simulink model "P_simple_sim_non_linear_model"  (R2015b)
settings: Solver=FixedStepAuto  StartTime=0.0  StopTime=t_f  FixedStep=0.005  RelTol=1e-3
values from neighbouring files (symbols this model uses):
  a = 0.3    [ICPtesting.m]    (also in LQR_controller_development.m = 0.0165; LQR_controller_development_new.m = 0.0165; RotationMatrixProperties.m; controller_params.m = 0.0165)
  b = 20*pi/180    (= 0.349065850399)    [LQR_controller_development.m]    (also in LQR_controller_development_new.m; RotationMatrixProperties.m = 0.3; controller_params.m)
  bp = 0.6    [LQR_controller_development.m]    (also in LQR_controller_development_new.m = 0.03; controller_params.m = 0.84111335)
  br = 0.3    [LQR_controller_development.m]    (also in LQR_controller_development_new.m = 0.03; controller_params.m = 0.246502067333)
  bw = 0.6    [LQR_controller_development.m]    (also in LQR_controller_development_new.m = 0.03; controller_params.m = 0.377213737333)
  bx = 10    [LQR_controller_development.m]    (also in LQR_controller_development_new.m = 12; controller_params.m = 7.95)
  by = 20    [LQR_controller_development.m]    (also in LQR_controller_development_new.m = 16; controller_params.m = 22.75)
  bz = 20    [LQR_controller_development.m]    (also in LQR_controller_development_new.m = 18; controller_params.m = 37.1)
  c = double(solve(cos(c_sym)*a-sin(c_sym)*lbx == 0,c_sym))    [LQR_controller_development.m]    (also in LQR_controller_development_new.m; RotationMatrixProperties.m = 0.3; controller_params.m = 8)
  dt = 0.02    [LQR_controller_development.m]    (also in LQR_controller_development_new.m = 0.05; controller_params.m = 0.05)
  Ixx = 0.015    [LQR_controller_development.m]    (also in LQR_controller_development_new.m; controller_params.m = 0.0098)
  Iyy = 0.035    [LQR_controller_development.m]    (also in LQR_controller_development_new.m; controller_params.m = 0.075)
  Izz = 0.035    [LQR_controller_development.m]    (also in LQR_controller_development_new.m; controller_params.m = 0.08)
  Kd = round(Kd,4)    [LQI_controller_development.m]    (also in LQR_controller_development.m; LQR_controller_development_new.m)
  lax = 0.15    [LQR_controller_development.m]    (also in LQR_controller_development_new.m; controller_params.m = 0.2)
  lay = 0.1    [LQR_controller_development.m]    (also in LQR_controller_development_new.m; controller_params.m)
  lbx = 0.12    [LQR_controller_development.m]    (also in LQR_controller_development_new.m; controller_params.m = 0.175)
  m = m*1.2    [LQI_controller_development.m]    (also in LQR_controller_development.m = 3; LQR_controller_development_new.m = 4; controller_params.m = 3.8)
  Tp_deadband = 0.2    [LQR_controller_development.m]    (also in LQR_controller_development_new.m = 0.1; controller_params.m = 0.05)
  Tp_min_input = 0.5    [LQR_controller_development.m]    (also in LQR_controller_development_new.m = 0.2; controller_params.m = 0.1)
  TpL = -140    [LQR_controller_development.m]    (also in LQR_controller_development_new.m = -22; controller_params.m = -8)
  TpU = 160    [LQR_controller_development.m]    (also in LQR_controller_development_new.m = 25; controller_params.m = 8)
  Ts_deadband = 0.2    [LQR_controller_development.m]    (also in LQR_controller_development_new.m = 0.1; controller_params.m = 0.05)
  Ts_min_input = 0.5    [LQR_controller_development.m]    (also in LQR_controller_development_new.m = 0.2; controller_params.m = 0.1)
  TsL = -70    [LQR_controller_development.m]    (also in LQR_controller_development_new.m = -14; controller_params.m = -4)
  TsU = 80    [LQR_controller_development.m]    (also in LQR_controller_development_new.m = 15; controller_params.m = 4)
undefined symbols (not defined in the file or in its folder): DiscIntNeverNeededParam
settings Model: Creator=meskupie  LastModifiedBy=meskupie

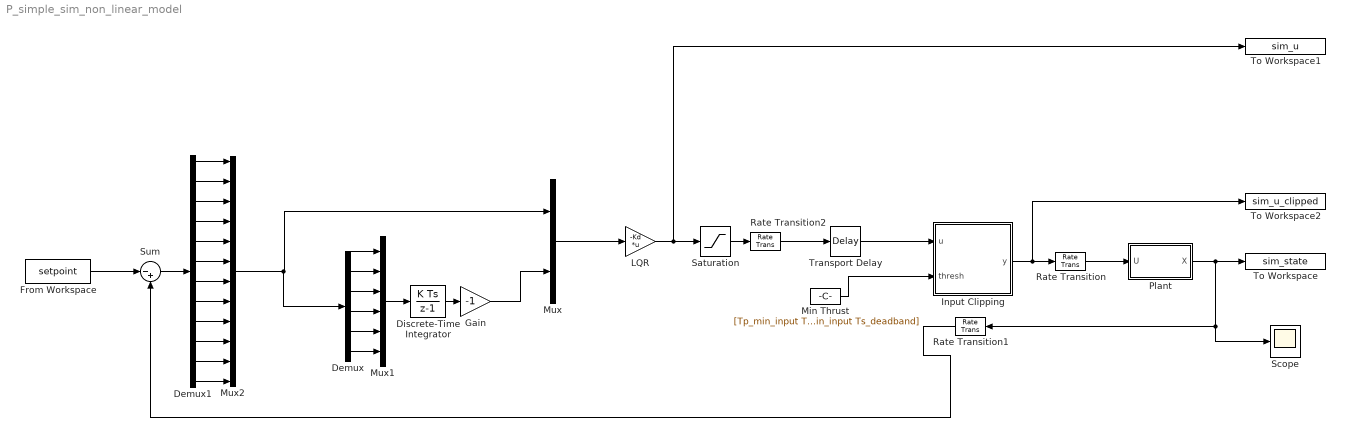
== system P_simple_sim_non_linear_model ==
  Demux : Demux  Outputs=12
  Demux1 : Demux  Outputs=12
  Discrete-Time Integrator : DiscreteIntegrator  InitialConditionSetting=State (most efficient)  SampleTime=dt  ICPrevOutput=DiscIntNeverNeededParam  ICPrevScaledInput=DiscIntNeverNeededParam
  From Workspace : FromWorkspace  VariableName=setpoint  SampleTime=dt
  Gain : Gain  Gain=-1
  Input Clipping : MATLAB Function  TreatAsAtomicUnit=on
  LQR : Gain  Gain=-Kd  Multiplication=Matrix(K*u)
  Min Thrust : Constant  Value=[Tp_min_input Tp_deadband Ts_min_input Ts_deadband]  SampleTime=-1
  Mux : Mux  Inputs=2
  Mux1 : Mux  Inputs=6
  Mux2 : Mux  Inputs=12
  Plant : Subsystem
  Rate Transition : RateTransition  OutPortSampleTimeOpt=Inherit
  Rate Transition1 : RateTransition  OutPortSampleTime=dt
  Rate Transition2 : RateTransition
  Saturation : Saturate  UpperLimit=[TpU TpU TpU TpU TsU TsU]  LowerLimit=[TpL TpL TpL TpL TsL TsL]
  Scope : Scope
  Sum : Sum  Inputs=|-+
  To Workspace : ToWorkspace  VariableName=sim_state  SaveFormat=Structure With Time  SampleTime=-1
  To Workspace1 : ToWorkspace  VariableName=sim_u  SaveFormat=Structure With Time  SampleTime=-1
  To Workspace2 : ToWorkspace  VariableName=sim_u_clipped  SaveFormat=Structure With Time  SampleTime=-1
  Transport Delay : TransportDelay  DelayTime=0.08
  wires:
  Mux2/1 -> Demux/1, Mux/1
  LQR/1 -> To Workspace1/1, Saturation/1
  Saturation/1 -> Rate Transition2/1
  Rate Transition/1 -> Plant/1(U)
  Plant/1(X) -> Scope/1, Rate Transition1/1, To Workspace/1
  Rate Transition1/1 -> Sum/2
  Min Thrust/1 -> Input Clipping/2(thresh)
  Input Clipping/1(y) -> To Workspace2/1, Rate Transition/1
  From Workspace/1 -> Sum/1
  Transport Delay/1 -> Input Clipping/1(u)
  Rate Transition2/1 -> Transport Delay/1
  Mux/1 -> LQR/1
  Demux/1 -> Mux1/1
  Demux/3 -> Mux1/2
  Demux/5 -> Mux1/3
  Demux/7 -> Mux1/4
  Demux/9 -> Mux1/5
  Demux/11 -> Mux1/6
  Mux1/1 -> Discrete-Time Integrator/1
  Discrete-Time Integrator/1 -> Gain/1
  Gain/1 -> Mux/2
  Sum/1 -> Demux1/1
  Demux1/2 -> Mux2/2
  Demux1/3 -> Mux2/3
  Demux1/4 -> Mux2/4
  Demux1/5 -> Mux2/5
  Demux1/6 -> Mux2/6
  Demux1/7 -> Mux2/7
  Demux1/8 -> Mux2/8
  Demux1/9 -> Mux2/9
  Demux1/10 -> Mux2/10
  Demux1/11 -> Mux2/11
  Demux1/12 -> Mux2/12
  Demux1/1 -> Mux2/1

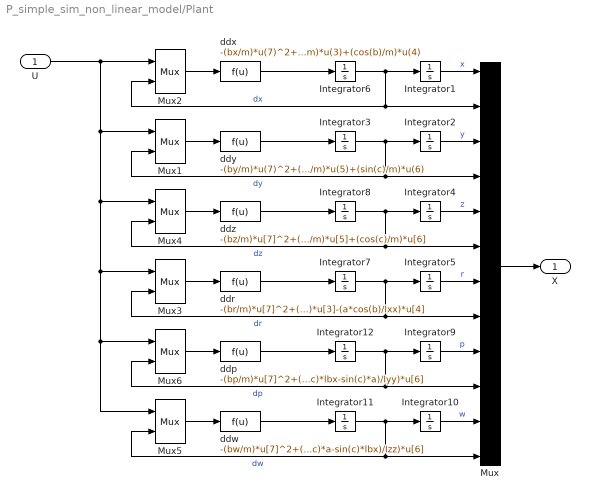
== system P_simple_sim_non_linear_model/Plant ==
  U : Inport
  Integrator{1..12} (12 alike) : Integrator
  Mux : Mux  Inputs=12
      settings: DisplayOption=signals
  Mux{1..6} (6 alike) : Mux  Inputs=2
  ddp : Fcn  Expr=-(bp/m)*u[7]^2+(a*cos(b)/Ixx)*u[1]-(a*cos(b)/Ixx)*u[2]+(a*cos(b)/Ixx)*u[3]-(a*cos(b)/Ixx)*u[4]-((cos(c)*lbx+sin(c)*a)/Iyy)*u[5]+((cos(c)*lbx-sin(c)*a)/Iyy)*u[6]
  ddr : Fcn  Expr=-(br/m)*u[7]^2+(a*cos(b)/Ixx)*u[1]+(a*cos(b)/Ixx)*u[2]-(a*cos(b)/Ixx)*u[3]-(a*cos(b)/Ixx)*u[4]
  ddw : Fcn  Expr=-(bw/m)*u[7]^2+((lay*cos(b)+lax*sin(b))/Izz)*u[1]-((lay*cos(b)+lax*sin(b))/Izz)*u[2]+((lay*cos(b)+lax*sin(b))/Izz)*u[3]-((lay*cos(b)+lax*sin(b))/Izz)*u[4]+((cos(c)*a-sin(c)*lbx)/Izz)*u[5]-((cos(c)*a-sin(c)*lbx)/Izz)*u[6]
  ddx : Fcn  Expr=-(bx/m)*u(7)^2+(cos(b)/m)*u(1)+(cos(b)/m)*u(2)+(cos(b)/m)*u(3)+(cos(b)/m)*u(4)
  ddy : Fcn  Expr=-(by/m)*u(7)^2+(sin(b)/m)*u(1)-(sin(b)/m)*u(2)-(sin(b)/m)*u(3)+(sin(b)/m)*u(4)-(sin(c)/m)*u(5)+(sin(c)/m)*u(6)
  ddz : Fcn  Expr=-(bz/m)*u[7]^2+(cos(c)/m)*u[5]+(cos(c)/m)*u[6]
  X : Outport
  wires:
  Mux2/1 -> ddx/1
  ddx/1 -> Integrator6/1
  Integrator6/1 -> Integrator1/1, Mux/2, Mux2/2  "dx"
  Mux1/1 -> ddy/1
  ddy/1 -> Integrator3/1
  Integrator3/1 -> Integrator2/1, Mux/4, Mux1/2  "dy"
  Mux4/1 -> ddz/1
  ddz/1 -> Integrator8/1
  Integrator8/1 -> Integrator4/1, Mux/6, Mux4/2  "dz"
  Mux3/1 -> ddr/1
  ddr/1 -> Integrator7/1
  Integrator7/1 -> Integrator5/1, Mux/8, Mux3/2  "dr"
  Mux6/1 -> ddp/1
  ddp/1 -> Integrator12/1
  Integrator12/1 -> Integrator9/1, Mux/10, Mux6/2  "dp"
  Mux5/1 -> ddw/1
  ddw/1 -> Integrator11/1
  Integrator11/1 -> Integrator10/1, Mux/12, Mux5/2  "dw"
  U/1 -> Mux5/1, Mux6/1, Mux3/1, Mux4/1, Mux1/1, Mux2/1
  Integrator1/1 -> Mux/1  "x"
  Integrator4/1 -> Mux/5  "z"
  Integrator2/1 -> Mux/3  "y"
  Integrator5/1 -> Mux/7  "r"
  Integrator9/1 -> Mux/9  "p"
  Integrator10/1 -> Mux/11  "w"
  Mux/1 -> X/1

== matlab function P_simple_sim_non_linear_model/Input Clipping ==
  data: u input; y output; thresh input
function y = fcn(u,thresh)

for i = 1:4
    if (u(i) > 0 && u(i) < thresh(1))
        if u(i) > thresh(2)
            u(i) = thresh(1);
        else
            u(i) = 0;
        end
    elseif (u(i) < 0 && u(i) > -thresh(1))
        if u(i) < -thresh(2)
            u(i) = -thresh(1);
        else
            u(i) = 0;
        end
    end
end
for i = 5:6
    if (u(i) > 0 && u(i) < thresh(3))
        if u(i) > thresh(4)
            u(i) = thresh(3);
        else
            u(i) = 0;
        end
    elseif (u(i) < 0 && u(i) > -thresh(2))
        if u(i) < -thresh(4)
            u(i) = -thresh(3);
        else
            u(i) = 0;
        end
    end
end
y = u;
